simulink model "Inverter"  (R2015b)
settings: Solver=ode23tb  StartTime=0.0  StopTime=3  RelTol=1e-5
libraries: powerlib x24, powerlib_meascontrol x5, simulink x3, pePwmGenerator x1
settings Model: Creator=Luis Mosquera  LastModifiedBy=MERT KARADENIZ
settings DataIOCC: SaveFormat=Array
settings DebuggingCC: AllowSymbolicDim=on
settings HardwareCC: ProdBitPerPointer=32  ProdLargestAtomicFloat=None  ProdIntDivRoundTo=Undefined  ProdEndianess=Unspecified  ProdWordSize=32  ProdHWDeviceType=32-bit Generic
settings GRTTargetCC: GeneratePreprocessorConditionals=Disable all
settings ConfigComp: CovModelRefEnable=Off
settings SimscapeCC: SimscapeNormalizeSystem=off
settings ConfigurationSet: Description=Simscape Multibody

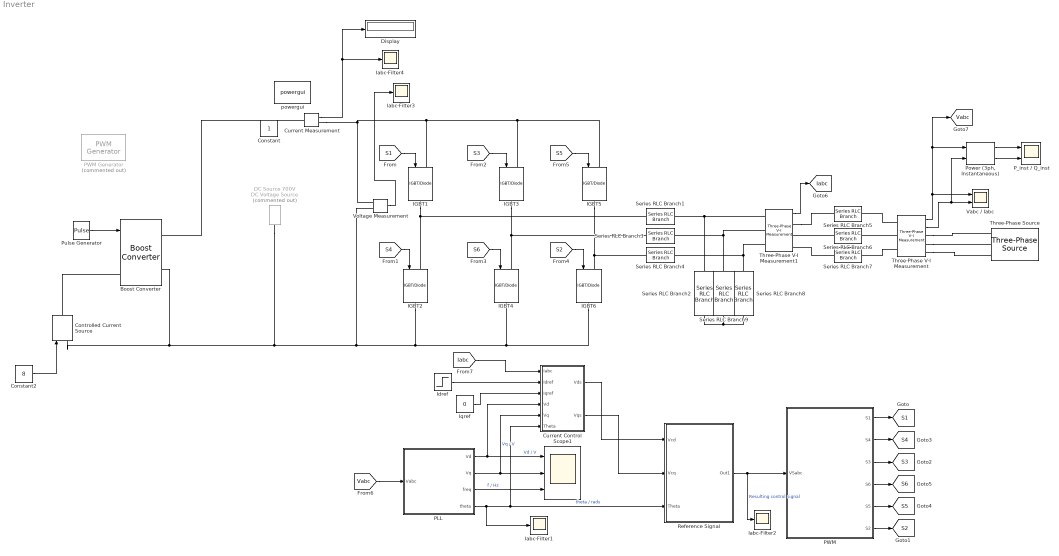
== system Inverter ==
  Boost Converter : powerlib/Power Electronics/Boost Converter  ModelType=Switching devices  Ron=1e-3  Rs=1e6  Cs=inf  Vforward=[0,0]  Ron_Diode=1e-3  Rs_Diode=1e6  Cs_Diode=inf  Vf_Diode=1e-3  Rs_CurrentSource=inf
  Constant2 : Constant  Value=8
  Controlled Current Source : powerlib/Electrical Sources/Controlled Current Source  Initialize=on  Source_Type=DC  Amplitude=0  Phase=0  Frequency=0  Measurements=None
  Current Control : Subsystem
  Current Measurement : powerlib/Measurements/Current Measurement  PhasorSimulation=off  OutputType=Complex  PSBequivalent=0
  DC Source 700V : powerlib/Electrical Sources/DC Voltage Source  Commented=on  Amplitude=700  Measurements=None
  Display : Display
  IGBT{1..6} (6 alike) : powerlib/Power Electronics/IGBT//Diode  Ron=1e-3  Rs=1e5  Cs=inf  Measurements=off
  Iabc-Filter{1..4} (4 alike) : Scope
  Idref : Step  Before=5  After=0  SampleTime=0
  Iqref : Constant  Value=0
  PLL : Subsystem
  PWM : Subsystem
  PWM Generator : pePwmGenerator/PWM Generator  Commented=on  CarrCount=Up  Tper=0.001  Ts=5e-5
  P_inst / Q_inst : Scope  NumInputPorts=2
  "Power (3ph, Instantaneous)" : powerlib_meascontrol/Measurements/Power (3ph, Instantaneous)
  Pulse Generator : DiscretePulseGenerator  PulseType=Time based  Period=1/5000  PulseWidth=20
  Reference Signal : Subsystem
  Scope1 : Scope  NumInputPorts=3
  Series RLC Branch1 : powerlib/Elements/Series RLC Branch  LConnTagsString=__new0  RConnTagsString=__new0  BranchType=L  Resistance=1  Inductance=2.5e-3  SetiL0=off  InitialCurrent=0  Capacitance=1e-6  Setx0=off  InitialVoltage=0  Measurements=None
  Series RLC Branch2 : powerlib/Elements/Series RLC Branch  LConnTagsString=__new0  RConnTagsString=__new0  BranchType=RC  Resistance=3.1*50  Inductance=1e-3  SetiL0=off  InitialCurrent=0  Capacitance=15e-6  Setx0=off  InitialVoltage=0  Measurements=None
  Series RLC Branch3 : powerlib/Elements/Series RLC Branch  LConnTagsString=__new0  RConnTagsString=__new0  BranchType=L  Resistance=1  Inductance=2.5e-3  SetiL0=off  InitialCurrent=0  Capacitance=1e-6  Setx0=off  InitialVoltage=0  Measurements=None
  Series RLC Branch4 : powerlib/Elements/Series RLC Branch  LConnTagsString=__new0  RConnTagsString=__new0  BranchType=L  Resistance=1  Inductance=2.5e-3  SetiL0=off  InitialCurrent=0  Capacitance=1e-6  Setx0=off  InitialVoltage=0  Measurements=None
  Series RLC Branch5 : powerlib/Elements/Series RLC Branch  LConnTagsString=__new0  RConnTagsString=__new0  BranchType=L  Resistance=1  Inductance=2e-3  SetiL0=off  InitialCurrent=0  Capacitance=1e-6  Setx0=off  InitialVoltage=0  Measurements=None
  Series RLC Branch6 : powerlib/Elements/Series RLC Branch  LConnTagsString=__new0  RConnTagsString=__new0  BranchType=L  Resistance=1  Inductance=2e-3  SetiL0=off  InitialCurrent=0  Capacitance=1e-6  Setx0=off  InitialVoltage=0  Measurements=None
  Series RLC Branch7 : powerlib/Elements/Series RLC Branch  LConnTagsString=__new0  RConnTagsString=__new0  BranchType=L  Resistance=1  Inductance=2e-3  SetiL0=off  InitialCurrent=0  Capacitance=1e-6  Setx0=off  InitialVoltage=0  Measurements=None
  Series RLC Branch8 : powerlib/Elements/Series RLC Branch  LConnTagsString=__new0  RConnTagsString=__new0  BranchType=RC  Resistance=3.1*50  Inductance=1e-3  SetiL0=off  InitialCurrent=0  Capacitance=15e-6  Setx0=off  InitialVoltage=0  Measurements=None
  Series RLC Branch9 : powerlib/Elements/Series RLC Branch  LConnTagsString=__new0  RConnTagsString=__new0  BranchType=RC  Resistance=3.1*50  Inductance=1e-3  SetiL0=off  InitialCurrent=0  Capacitance=15e-6  Setx0=off  InitialVoltage=0  Measurements=None
  Three-Phase V-I Measurement : powerlib/Measurements/Three-Phase V-I Measurement  VoltageMeasurement=phase-to-ground  SetLabelV=off  LabelV=Vabc  Vpu=off  VpuLL=off  CurrentMeasurement=yes  SetLabelI=off  LabelI=Iabc  Ipu=off  Pbase=100e6  Vbase=500e3  OutputType=Complex  PhasorSimulation=off  PSBequivalent=0
  Three-Phase V-I Measurement1 : powerlib/Measurements/Three-Phase V-I Measurement  VoltageMeasurement=no  SetLabelV=off  LabelV=Vabc  Vpu=off  VpuLL=off  CurrentMeasurement=yes  SetLabelI=off  LabelI=Iabc  Ipu=off  Pbase=100e6  Vbase=500e3  OutputType=Complex  PhasorSimulation=off  PSBequivalent=0
  Three-Phase Source : powerlib/Electrical Sources/Three-Phase Source  InternalConnection=Yg  VoltagePhases=off  Voltage=400  PhaseAngle=0  Voltage_phases=[25e3 25e3 25e3]/sqrt(3)  PhaseAngles_phases=[0 -120 +120]  Frequency=50  NonIdealSource=off  SpecifyImpedance=off  Resistance=0.48  Inductance=250e-6  ShortCircuitLevel=100e6  BaseVoltage=400  XRratio=7  BusType=swing  Pref=0  Qref=0  Prefabc=[10e3, 10e3, 10e3]  Qrefabc=[0, 0, 0]  Qmin=-inf  Qmax=inf
  Vabc / Iabc : Scope  NumInputPorts=2
  Voltage Measurement : powerlib/Measurements/Voltage Measurement  PhasorSimulation=off  OutputType=Complex  PSBequivalent=0
  powergui : powerlib/powergui  Priority=1  SimulationMode=Discrete  SampleTime=1e-6  frequency=60  Iterations=50  frequencyindice=50  Pbase=100e6  ErrMax=1e-4  UnitsV=kV  UnitsW=MW  buscounter=0  FunctionMessages=off  echomessages=off  EnableUseOfTLC=off  CurrentSourceSwitches=off  DisableSnubberDevices=on  DisableRonSwitches=on  DisableVfSwitches=on  DisplayEquations=on  SolverType=Tustin/Backward Euler (TBE)  Interpol=off  ExternalGateDelay=off  methode=off  Ts=100  x0status=blocks  SPID=on  SwTol=0  HookPort=off  RestoreLinks=warning  ResistiveCurrentMeasurement=off  Frange=[0:2:500]  Ylog=off  Xlog=on  ShowGrid=off  save=off  variable=ZData  structure=0  ZoomFFT=off  StartTime=0.0  cycles=1  DisplayStyle=1  fundamental=60  FreqAxis=off  MaxFrequency=1000  frequencyindicesteady=1  RmsSteady=1  display=off
  Constant : Constant  IOType=siggen
  tag scope: Iabc=global, S1=global, S2=global, S3=global, S4=global, S5=global, S6=global, Vabc=global
  wires:
  [S1] -> IGBT1/1
  [S4] -> IGBT2/1
  [S3] -> IGBT3/1
  [S6] -> IGBT4/1
  [S5] -> IGBT5/1
  [S2] -> IGBT6/1
  PWM/2(S4) -> [S4]
  PWM/4(S6) -> [S6]
  PWM/1(S1) -> [S1]
  PWM/3(S3) -> [S3]
  PWM/5(S5) -> [S5]
  PWM/6(S2) -> [S2]
  Three-Phase V-I Measurement/2 -> "Power (3ph, Instantaneous)"/2, Vabc / Iabc/2
  Three-Phase V-I Measurement/1 -> "Power (3ph, Instantaneous)"/1, [Vabc], Vabc / Iabc/1
  [Vabc] -> PLL/1(Vabc)
  PLL/1(Vd) -> Scope1/1, Current Control/4(Vd)  "Vd / V"
  PLL/2(Vq) -> Scope1/2, Current Control/5(Vq)  "Vq / V"
  PLL/3(freq) -> Scope1/3  "f / Hz"
  PLL/4(theta) -> Reference Signal/3(Theta), Current Control/6(Theta), Iabc-Filter1/1  "theta / rads"
  Reference Signal/1(Out1) -> Iabc-Filter2/1, PWM/1(VSabc)  "Resulting control signal"
  Three-Phase V-I Measurement1/1 -> [Iabc]
  [Iabc] -> Current Control/1(Iabc)
  Idref/1 -> Current Control/2(Idref)
  Iqref/1 -> Current Control/3(Iqref)
  Current Control/2(Vqs) -> Reference Signal/2(Vcq)
  "Power (3ph, Instantaneous)"/1 -> P_inst / Q_inst/1
  "Power (3ph, Instantaneous)"/2 -> P_inst / Q_inst/2
  Current Control/1(Vds) -> Reference Signal/1(Vcd)
  Voltage Measurement/1 -> Iabc-Filter3/1
  Current Measurement/1 -> Display/1, Iabc-Filter4/1
  Constant2/1 -> Controlled Current Source/1
  Pulse Generator/1 -> Boost Converter/1
  connections:
  IGBT1/RConn1 -- IGBT2/LConn1 -- Series RLC Branch1/LConn1
  IGBT3/RConn1 -- Series RLC Branch3/LConn1 -- IGBT4/LConn1
  IGBT5/RConn1 -- Series RLC Branch4/LConn1 -- IGBT6/LConn1
  Voltage Measurement/LConn1 -- Current Measurement/RConn1 -- IGBT5/LConn1 -- IGBT3/LConn1 -- IGBT1/LConn1
  Series RLC Branch2/LConn1 -- Three-Phase V-I Measurement1/LConn1 -- Series RLC Branch1/RConn1
  Series RLC Branch9/LConn1 -- Series RLC Branch3/RConn1 -- Three-Phase V-I Measurement1/LConn2
  Series RLC Branch8/LConn1 -- Three-Phase V-I Measurement1/LConn3 -- Series RLC Branch4/RConn1
  Series RLC Branch2/RConn1 -- Series RLC Branch9/RConn1 -- Series RLC Branch8/RConn1
  Series RLC Branch7/LConn1 -- Three-Phase V-I Measurement1/RConn3
  Series RLC Branch6/LConn1 -- Three-Phase V-I Measurement1/RConn2
  Three-Phase V-I Measurement1/RConn1 -- Series RLC Branch5/LConn1
  Three-Phase V-I Measurement/LConn1 -- Series RLC Branch5/RConn1
  Three-Phase V-I Measurement/LConn2 -- Series RLC Branch6/RConn1
  Three-Phase V-I Measurement/LConn3 -- Series RLC Branch7/RConn1
  Three-Phase V-I Measurement/RConn1 -- Three-Phase Source/RConn1
  Three-Phase V-I Measurement/RConn2 -- Three-Phase Source/RConn2
  Three-Phase V-I Measurement/RConn3 -- Three-Phase Source/RConn3
  Controlled Current Source/RConn1 -- Boost Converter/LConn1
  Voltage Measurement/LConn2 -- Controlled Current Source/LConn1 -- Boost Converter/RConn2 -- DC Source 700V/LConn1 -- IGBT6/RConn1 -- IGBT4/RConn1 -- IGBT2/RConn1
  Current Measurement/LConn1 -- Boost Converter/RConn1

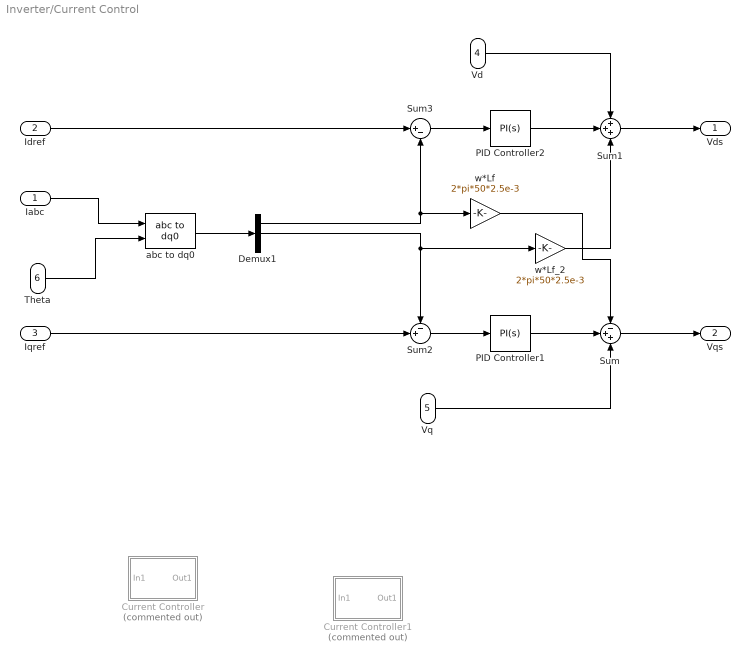
== system Inverter/Current Control ==
  Iabc : Inport
  Idref : Inport  Port=2
  Iqref : Inport  Port=3
  Vd : Inport  Port=4
  Vq : Inport  Port=5
  Theta : Inport  Port=6
  Current Controller : Subsystem  Commented=on
  Current Controller1 : Subsystem  Commented=on
  Demux1 : Demux  Outputs=3
  PID Controller1 : simulink/Continuous/PID Controller  Controller=PI  TimeDomain=Continuous-time  SampleTime=-1  IntegratorMethod=Forward Euler  FilterMethod=Forward Euler  Form=Ideal  UseFilter=on  ControllerParametersSource=internal  P=((2.5e-3+2e-3)*((2*pi*500)+(2*pi*100)))  I=(2.5e-3+2e-3)*(2*pi*500)*(2*pi*100)/100  D=0  N=100  InitialConditionSource=internal  InitialConditionForIntegrator=0  InitialConditionForFilter=0  ExternalReset=none  LimitOutput=on  UpperSaturationLimit=350  LowerSaturationLimit=-350  LinearizeAsGain=on  AntiWindupMode=back-calculation  Kb=1  TrackingMode=off  Kt=1  PParamMin=[]  PParamMax=[]  IParamMin=[]  IParamMax=[]  DParamMin=[]  DParamMax=[]  NParamMin=[]  NParamMax=[]  KbParamMin=[]  KbParamMax=[]  KtParamMin=[]  KtParamMax=[]  POutMin=[]  POutMax=[]  IOutMin=[]  IOutMax=[]  DOutMin=[]  DOutMax=[]  NOutMin=[]  NOutMax=[]  KbOutMin=[]  KbOutMax=[]  KtOutMin=[]  KtOutMax=[]  IntegratorOutMin=[]  IntegratorOutMax=[]  FilterOutMin=[]  FilterOutMax=[]  SumOutMin=[]  SumOutMax=[]  SumI1OutMin=[]  SumI1OutMax=[]  SumI2OutMin=[]  SumI2OutMax=[]  SumI3OutMin=[]  SumI3OutMax=[]  SumDOutMin=[]  SumDOutMax=[]  SaturationOutMin=[]  SaturationOutMax=[]  IntegratorContinuousStateAttributes=''  IntegratorStateMustResolveToSignalObject=off  IntegratorRTWStateStorageClass=Auto  FilterContinuousStateAttributes=''  FilterStateMustResolveToSignalObject=off  FilterRTWStateStorageClass=Auto  DifferentiatorICPrevScaledInput=0  DifferentiatorOutMin=[]  DifferentiatorOutMax=[]
  PID Controller2 : simulink/Continuous/PID Controller  Controller=PI  TimeDomain=Continuous-time  SampleTime=-1  IntegratorMethod=Forward Euler  FilterMethod=Forward Euler  Form=Ideal  UseFilter=on  ControllerParametersSource=internal  P=((2.5e-3+2e-3)*((2*pi*500)+(2*pi*100)))  I=(2.5e-3+2e-3)*(2*pi*500)*(2*pi*100)/100  D=0  N=100  InitialConditionSource=internal  InitialConditionForIntegrator=0  InitialConditionForFilter=0  ExternalReset=none  LimitOutput=on  UpperSaturationLimit=350  LowerSaturationLimit=-350  LinearizeAsGain=on  AntiWindupMode=back-calculation  Kb=1  TrackingMode=off  Kt=1  PParamMin=[]  PParamMax=[]  IParamMin=[]  IParamMax=[]  DParamMin=[]  DParamMax=[]  NParamMin=[]  NParamMax=[]  KbParamMin=[]  KbParamMax=[]  KtParamMin=[]  KtParamMax=[]  POutMin=[]  POutMax=[]  IOutMin=[]  IOutMax=[]  DOutMin=[]  DOutMax=[]  NOutMin=[]  NOutMax=[]  KbOutMin=[]  KbOutMax=[]  KtOutMin=[]  KtOutMax=[]  IntegratorOutMin=[]  IntegratorOutMax=[]  FilterOutMin=[]  FilterOutMax=[]  SumOutMin=[]  SumOutMax=[]  SumI1OutMin=[]  SumI1OutMax=[]  SumI2OutMin=[]  SumI2OutMax=[]  SumI3OutMin=[]  SumI3OutMax=[]  SumDOutMin=[]  SumDOutMax=[]  SaturationOutMin=[]  SaturationOutMax=[]  IntegratorContinuousStateAttributes=''  IntegratorStateMustResolveToSignalObject=off  IntegratorRTWStateStorageClass=Auto  FilterContinuousStateAttributes=''  FilterStateMustResolveToSignalObject=off  FilterRTWStateStorageClass=Auto  DifferentiatorICPrevScaledInput=0  DifferentiatorOutMin=[]  DifferentiatorOutMax=[]
  Sum : Sum  Inputs=-++
  Sum1 : Sum  Inputs=+++
  Sum2 : Sum  Inputs=-+|
  Sum3 : Sum  Inputs=|+-
  abc to dq0 : powerlib_meascontrol/Transformations/abc to dq0  Alignment=90 degrees behind phase A axis
  w*Lf : Gain  Gain=2*pi*50*2.5e-3
  w*Lf_2 : Gain  Gain=2*pi*50*2.5e-3
  Vds : Outport
  Vqs : Outport  Port=2
  wires:
  Idref/1 -> Sum3/1
  Demux1/1 -> w*Lf/1, Sum3/2
  Iqref/1 -> Sum2/2
  Demux1/2 -> w*Lf_2/1, Sum2/1
  Sum3/1 -> PID Controller2/1
  Sum2/1 -> PID Controller1/1
  PID Controller2/1 -> Sum1/2
  Vd/1 -> Sum1/1
  Vq/1 -> Sum/3
  PID Controller1/1 -> Sum/2
  w*Lf_2/1 -> Sum1/3
  w*Lf/1 -> Sum/1
  Sum1/1 -> Vds/1
  Sum/1 -> Vqs/1
  Iabc/1 -> abc to dq0/1
  Theta/1 -> abc to dq0/2
  abc to dq0/1 -> Demux1/1

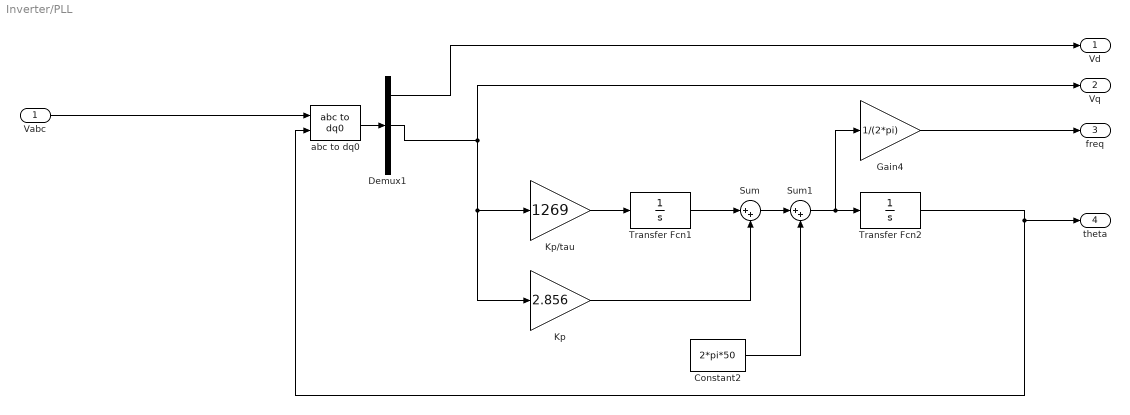
== system Inverter/PLL ==
  Vabc : Inport
  Constant2 : Constant  Value=2*pi*50
  Demux1 : Demux  Outputs=3
  Gain4 : Gain  Gain=1/(2*pi)
  Kp : Gain  Gain=2.856
  Kp/tau : Gain  Gain=1269
  Sum : Sum  Inputs=|++
  Sum1 : Sum  Inputs=|++
  Transfer Fcn1 : TransferFcn  Denominator=[1 0]
  Transfer Fcn2 : TransferFcn  Denominator=[1 0]
  abc to dq0 : powerlib_meascontrol/Transformations/abc to dq0  Alignment=90 degrees behind phase A axis
  Vd : Outport
  Vq : Outport  Port=2
  freq : Outport  Port=3
  theta : Outport  Port=4
  wires:
  Constant2/1 -> Sum1/2
  Sum1/1 -> Gain4/1, Transfer Fcn2/1
  Sum/1 -> Sum1/1
  Transfer Fcn1/1 -> Sum/1
  Kp/1 -> Sum/2
  Kp/tau/1 -> Transfer Fcn1/1
  Transfer Fcn2/1 -> abc to dq0/2, theta/1
  Gain4/1 -> freq/1
  Vabc/1 -> abc to dq0/1
  Demux1/2 -> Vq/1, Kp/tau/1, Kp/1
  Demux1/1 -> Vd/1
  abc to dq0/1 -> Demux1/1

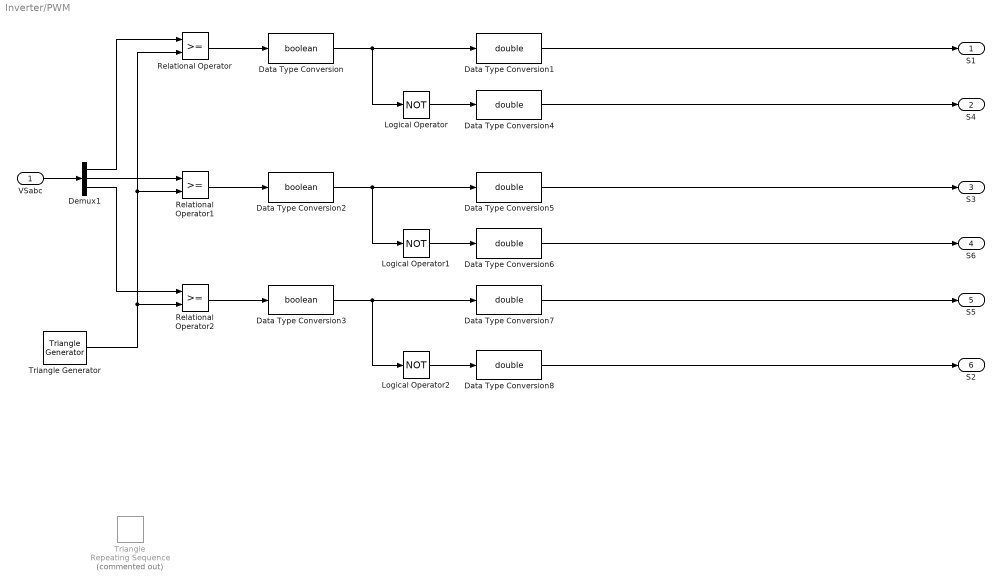
== system Inverter/PWM ==
  VSabc : Inport
  Data Type Conversion : DataTypeConversion  OutDataTypeStr=boolean
  Data Type Conversion{1,4..8} (6 alike) : DataTypeConversion  OutDataTypeStr=double
  Data Type Conversion2 : DataTypeConversion  OutDataTypeStr=boolean
  Data Type Conversion3 : DataTypeConversion  OutDataTypeStr=boolean
  Demux1 : Demux  Outputs=3
  Logical Operator : Logic  Operator=NOT  AllPortsSameDT=off  OutDataTypeStr=boolean
  Logical Operator1 : Logic  Operator=NOT  AllPortsSameDT=off  OutDataTypeStr=boolean
  Logical Operator2 : Logic  Operator=NOT  AllPortsSameDT=off  OutDataTypeStr=boolean
  Relational Operator : RelationalOperator  OutDataTypeStr=boolean
  Relational Operator1 : RelationalOperator  OutDataTypeStr=boolean
  Relational Operator2 : RelationalOperator  OutDataTypeStr=boolean
  Triangle : simulink/Sources/Repeating Sequence  Commented=on  rep_seq_t=[0 1/5000/4 3/5000/4 1/5000]  rep_seq_y=[0 1 -1 0]
  Triangle Generator : powerlib_meascontrol/Pulse & Signal Generators/Triangle Generator  Freq=5000  Phase=0  Ts=0
  S1 : Outport
  S4 : Outport  Port=2
  S3 : Outport  Port=3
  S6 : Outport  Port=4
  S5 : Outport  Port=5
  S2 : Outport  Port=6
  wires:
  VSabc/1 -> Demux1/1
  Logical Operator2/1 -> Data Type Conversion8/1
  Demux1/1 -> Relational Operator/1
  Triangle Generator/1 -> Relational Operator/2, Relational Operator1/2, Relational Operator2/2
  Data Type Conversion3/1 -> Logical Operator2/1, Data Type Conversion7/1
  Data Type Conversion2/1 -> Logical Operator1/1, Data Type Conversion5/1
  Logical Operator1/1 -> Data Type Conversion6/1
  Logical Operator/1 -> Data Type Conversion4/1
  Relational Operator2/1 -> Data Type Conversion3/1
  Relational Operator1/1 -> Data Type Conversion2/1
  Demux1/2 -> Relational Operator1/1
  Demux1/3 -> Relational Operator2/1
  Data Type Conversion/1 -> Data Type Conversion1/1, Logical Operator/1
  Relational Operator/1 -> Data Type Conversion/1
  Data Type Conversion1/1 -> S1/1
  Data Type Conversion4/1 -> S4/1
  Data Type Conversion5/1 -> S3/1
  Data Type Conversion6/1 -> S6/1
  Data Type Conversion7/1 -> S5/1
  Data Type Conversion8/1 -> S2/1

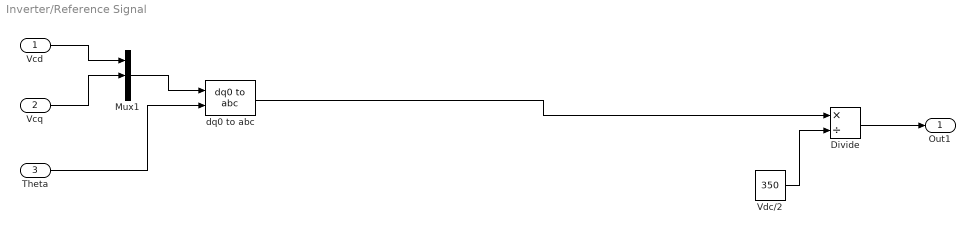
== system Inverter/Reference Signal ==
  Vcd : Inport
  Vcq : Inport  Port=2
  Theta : Inport  Port=3
  Divide : Product  Inputs=*/
  Mux1 : Mux  Inputs=3
  Vdc/2 : Constant  Value=350
  dq0 to abc : powerlib_meascontrol/Transformations/dq0 to abc  Alignment=90 degrees behind phase A axis
  Out1 : Outport
  wires:
  Vdc/2/1 -> Divide/2
  Vcd/1 -> Mux1/1
  Vcq/1 -> Mux1/2
  Theta/1 -> dq0 to abc/2
  Mux1/1 -> dq0 to abc/1
  Divide/1 -> Out1/1
  dq0 to abc/1 -> Divide/1

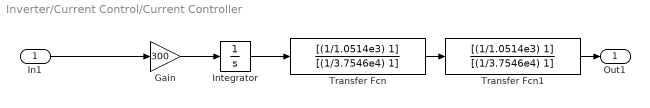
== system Inverter/Current Control/Current Controller ==
  In1 : Inport
  Gain : Gain  Gain=300
  Integrator : Integrator
  Transfer Fcn : TransferFcn  Numerator=[(1/1.0514e3) 1]  Denominator=[(1/3.7546e4) 1]
  Transfer Fcn1 : TransferFcn  Numerator=[(1/1.0514e3) 1]  Denominator=[(1/3.7546e4) 1]
  Out1 : Outport
  wires:
  Transfer Fcn1/1 -> Out1/1
  Transfer Fcn/1 -> Transfer Fcn1/1
  Gain/1 -> Integrator/1
  Integrator/1 -> Transfer Fcn/1
  In1/1 -> Gain/1

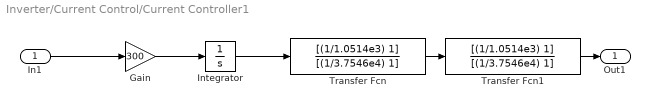
== system Inverter/Current Control/Current Controller1 ==
  In1 : Inport
  Gain : Gain  Gain=300
  Integrator : Integrator
  Transfer Fcn : TransferFcn  Numerator=[(1/1.0514e3) 1]  Denominator=[(1/3.7546e4) 1]
  Transfer Fcn1 : TransferFcn  Numerator=[(1/1.0514e3) 1]  Denominator=[(1/3.7546e4) 1]
  Out1 : Outport
  wires:
  Transfer Fcn1/1 -> Out1/1
  Transfer Fcn/1 -> Transfer Fcn1/1
  Gain/1 -> Integrator/1
  Integrator/1 -> Transfer Fcn/1
  In1/1 -> Gain/1
